simulink library "tqd"  (R2021b)
settings: Solver=VariableStepAuto  StartTime=0.0  StopTime=10.0  RelTol=1e-3
undefined symbols (not defined in the file or in its folder): ATQD_AccelLimitInRange_X_rpm, ATQD_AccelLimitInRange_Y_Nm, ATQD_AccelLimitOvrKi_X_Nm, ATQD_AccelLimitOvrKp_X_Nm, ATQD_BOSMapD_X_rpm, ATQD_BOSMapD_Y_pct, ATQD_BOSMapR_X_rpm, ATQD_BOSMapR_Y_pct, ATQD_HVBCurrSmooth_X_A, ATQD_LHMTqMapDLC_X_rpm, ATQD_LHMTqMapDLC_Y_pct, ATQD_LHMTqMapRLC_X_rpm, ATQD_LHMTqMapRLC_Y_pct, ATQD_NormalMapDLC_X_rpm, ATQD_NormalMapDLC_Y_pct, ATQD_NormalTqDecSR_X_rpm, ATQD_NormalTqDecSR_Y_Nm, ATQD_NormalTqIncSR_X_rpm, ATQD_NormalTqIncSR_Y_Nm, ATQD_OPDMapRLC_X_rpm, ATQD_OPDMapRLC_Y_pct, ATQD_RollRegTorReq_X_rpm, ATQD_RollRegTorReq_Y_enum, ATQD_VehSpdLimitInRange_X_rpm, ATQD_VehSpdLimitInRange_Y_Nm, ATQD_VehSpdLimitOvrKi_X_Nm, ATQD_VehSpdLimitOvrKp_X_Nm, EIGHT_INT, ENUM_BRAKEPEDAL_PRESSED, ENUM_BRAKEPEDAL_RELEASED, ENUM_COMBOKEY_DOWN, ENUM_COMBOKEY_M1, ENUM_COMBOKEY_M2, ENUM_COMBOKEY_NONE, ENUM_COMBOKEY_RKNEE, ENUM_COMBOKEY_STOPLV, ENUM_COMBOKEY_UP, ENUM_CP2VKNEEREQ_REQUEST, ENUM_CP2VNLVREQ_LEVEL1, ENUM_CP2VNLVREQ_LEVEL2, ENUM_CP2VNLVREQ_LOWER, ENUM_CP2VNLVREQ_STOPLV, ENUM_CP2VNLVREQ_UPPER, ENUM_CREEPIND_DISABLE, ENUM_CREEPIND_READY, ENUM_CREEPIND_RUNNING, ENUM_CREEPIND_WARNING, ENUM_DRIVELINERELEASE_RELEASE, ENUM_EBSTORQUERWQ_LIMIT, ENUM_EBSTORQUERWQ_TORQUE, ENUM_ECPVCUDRM_CONFORT, ENUM_ECPVCUDRM_ECO, ENUM_ECPVCUDRM_NORMAL, ENUM_ECPVCUDRM_NOTAVAILABLE, ENUM_EMTqModeDrvBrk_Accel, ENUM_EMTqModeDrvBrk_Brake, ENUM_EMTqModeDrvBrk_Coast, ENUM_ETC2ACTDRIVEDIR_BACKWARD, ENUM_ETC2ACTDRIVEDIR_FORWARD, ENUM_ETC2ACTDRIVEDIR_STILL ... (+341)
libraries: simulink x109, hcu_lib x67
(part 13 of 13)

== stateflow chart tqd/TQD/OutpConvert/Buzzer Request/Combo Key Flasher/Chart ==
  state init
    en:
    time_cnt = ZERO_INT;
    ON_flg = TRUE;
    OFF_flg = FALSE;
    out = FALSE;
    CycleCnt_cnt = FALSE;
  state OFF
    en:
    out = FALSE;
    time_cnt = ZERO_INT;
    OFF -> (junction 38) [order 1]
    (junction 38) -> OFF : {time_cnt = time_cnt + ZERO_INT;}
  state ON
    en:
    out = TRUE;
    time_cnt = ZERO_INT;
    du:
    time_cnt = time_cnt + ONE_INT;
  state WAIT
    en:
    out = FALSE;
    time_cnt = ZERO_INT;
    du:
    time_cnt = time_cnt + ONE_INT;
  (default) -> init
  init -> (junction 57)
  (junction 57) -> ON : [ON_flg && VSCP_FlasherEn_flg]
  OFF -> (junction 46) [order 2] : [time_cnt > OFF_cnt]
  (junction 46) -> (junction 47) : {time_cnt = ZERO_INT;
      |  ON_flg = TRUE;
      |  OFF_flg = FALSE;
      |  CycleCnt_cnt = CycleCnt_cnt +ONE_INT;}
  (junction 47) -> ON : [ON_flg]
  ON -> (junction 44) : [time_cnt > ON_cnt]
  (junction 44) -> (junction 42) : {time_cnt = ZERO_INT;
      |  ON_flg = FALSE;
      |  OFF_flg = TRUE;}
  (junction 42) -> OFF : [OFF_flg]
  OFF -> (junction 66) [order 1] : [time_cnt > OFF_cnt && CycleCnt_cnt >= Cycle_cnt]
  (junction 66) -> WAIT : {time_cnt = ZERO_INT;}
  (junction 62) -> ON : {time_cnt = ZERO_INT;
      |  ON_flg = TRUE;
      |  OFF_flg = FALSE;
      |  CycleCnt_cnt = ZERO_INT;}
  WAIT -> (junction 62) : [time_cnt >= WAIT_cnt && VSCP_FlasherEn_flg]
  data: ON_cnt input; OFF_cnt input; WAIT_cnt input; Cycle_cnt input; out output boolean; time_cnt local uint8; OFF_flg local boolean; ON_flg local boolean; CycleCnt_cnt local uint8; VSCP_FlasherEn_flg input; FALSE parameter; TRUE parameter; ONE_INT parameter; ZERO_INT parameter

== stateflow chart tqd/TQD/OutpConvert/Buzzer Request/Parking Protect Flasher/Chart ==
  state init
    en:
    time_cnt = ZERO_INT;
    ON_flg = TRUE;
    OFF_flg = FALSE;
    out = FALSE;
    CycleCnt_cnt = FALSE;
  state OFF
    en:
    out = FALSE;
    time_cnt = ZERO_INT;
    OFF -> (junction 38) [order 1]
    (junction 38) -> OFF : {time_cnt = time_cnt + ZERO_INT;}
  state ON
    en:
    out = TRUE;
    time_cnt = ZERO_INT;
    du:
    time_cnt = time_cnt + ONE_INT;
  state WAIT
    en:
    out = FALSE;
    time_cnt = ZERO_INT;
    du:
    time_cnt = time_cnt + ONE_INT;
  (default) -> init
  init -> (junction 57)
  (junction 57) -> ON : [ON_flg && VSCP_FlasherEn_flg]
  OFF -> (junction 46) [order 2] : [time_cnt > OFF_cnt]
  (junction 46) -> (junction 47) : {time_cnt = ZERO_INT;
      |  ON_flg = TRUE;
      |  OFF_flg = FALSE;
      |  CycleCnt_cnt = CycleCnt_cnt +ONE_INT;}
  (junction 47) -> ON : [ON_flg]
  ON -> (junction 44) : [time_cnt > ON_cnt]
  (junction 44) -> (junction 42) : {time_cnt = ZERO_INT;
      |  ON_flg = FALSE;
      |  OFF_flg = TRUE;}
  (junction 42) -> OFF : [OFF_flg]
  OFF -> (junction 66) [order 1] : [time_cnt > OFF_cnt && CycleCnt_cnt >= Cycle_cnt]
  (junction 66) -> WAIT : {time_cnt = ZERO_INT;}
  (junction 62) -> ON : {time_cnt = ZERO_INT;
      |  ON_flg = TRUE;
      |  OFF_flg = FALSE;
      |  CycleCnt_cnt = ZERO_INT;}
  WAIT -> (junction 62) : [time_cnt >= WAIT_cnt && VSCP_FlasherEn_flg]
  data: ON_cnt input; OFF_cnt input; WAIT_cnt input; Cycle_cnt input; out output boolean; time_cnt local uint8; OFF_flg local boolean; ON_flg local boolean; CycleCnt_cnt local uint8; VSCP_FlasherEn_flg input; FALSE parameter; TRUE parameter; ONE_INT parameter; ZERO_INT parameter

== stateflow chart tqd/TQD/OutpConvert/Buzzer Request/Power Up Fail Flasher/Chart ==
  state init
    en:
    time_cnt = ZERO_INT;
    ON_flg = TRUE;
    OFF_flg = FALSE;
    out = FALSE;
    CycleCnt_cnt = FALSE;
  state OFF
    en:
    out = FALSE;
    time_cnt = ZERO_INT;
    OFF -> (junction 38) [order 1]
    (junction 38) -> OFF : {time_cnt = time_cnt + ZERO_INT;}
  state ON
    en:
    out = TRUE;
    time_cnt = ZERO_INT;
    du:
    time_cnt = time_cnt + ONE_INT;
  state WAIT
    en:
    out = FALSE;
    time_cnt = ZERO_INT;
    du:
    time_cnt = time_cnt + ONE_INT;
  (default) -> init
  init -> (junction 57)
  (junction 57) -> ON : [ON_flg && VSCP_FlasherEn_flg]
  OFF -> (junction 46) [order 2] : [time_cnt > OFF_cnt]
  (junction 46) -> (junction 47) : {time_cnt = ZERO_INT;
      |  ON_flg = TRUE;
      |  OFF_flg = FALSE;
      |  CycleCnt_cnt = CycleCnt_cnt +ONE_INT;}
  (junction 47) -> ON : [ON_flg]
  ON -> (junction 44) : [time_cnt > ON_cnt]
  (junction 44) -> (junction 42) : {time_cnt = ZERO_INT;
      |  ON_flg = FALSE;
      |  OFF_flg = TRUE;}
  (junction 42) -> OFF : [OFF_flg]
  OFF -> (junction 66) [order 1] : [time_cnt > OFF_cnt && CycleCnt_cnt >= Cycle_cnt]
  (junction 66) -> WAIT : {time_cnt = ZERO_INT;}
  (junction 62) -> ON : {time_cnt = ZERO_INT;
      |  ON_flg = TRUE;
      |  OFF_flg = FALSE;
      |  CycleCnt_cnt = ZERO_INT;}
  WAIT -> (junction 62) : [time_cnt >= WAIT_cnt && VSCP_FlasherEn_flg]
  data: ON_cnt input; OFF_cnt input; WAIT_cnt input; Cycle_cnt input; out output boolean; time_cnt local uint8; OFF_flg local boolean; ON_flg local boolean; CycleCnt_cnt local uint8; VSCP_FlasherEn_flg input; FALSE parameter; TRUE parameter; ONE_INT parameter; ZERO_INT parameter

== stateflow chart tqd/TQD/OutpConvert/Buzzer Request/Power Up Finished Flasher/Chart ==
  state init
    en:
    time_cnt = ZERO_INT;
    ON_flg = TRUE;
    OFF_flg = FALSE;
    out = FALSE;
    CycleCnt_cnt = FALSE;
  state OFF
    en:
    out = FALSE;
    time_cnt = ZERO_INT;
    OFF -> (junction 38) [order 1]
    (junction 38) -> OFF : {time_cnt = time_cnt + ZERO_INT;}
  state ON
    en:
    out = TRUE;
    time_cnt = ZERO_INT;
    du:
    time_cnt = time_cnt + ONE_INT;
  state WAIT
    en:
    out = FALSE;
    time_cnt = ZERO_INT;
    du:
    time_cnt = time_cnt + ONE_INT;
  (default) -> init
  init -> (junction 57)
  (junction 57) -> ON : [ON_flg && VSCP_FlasherEn_flg]
  OFF -> (junction 46) [order 2] : [time_cnt > OFF_cnt]
  (junction 46) -> (junction 47) : {time_cnt = ZERO_INT;
      |  ON_flg = TRUE;
      |  OFF_flg = FALSE;
      |  CycleCnt_cnt = CycleCnt_cnt +ONE_INT;}
  (junction 47) -> ON : [ON_flg]
  ON -> (junction 44) : [time_cnt > ON_cnt]
  (junction 44) -> (junction 42) : {time_cnt = ZERO_INT;
      |  ON_flg = FALSE;
      |  OFF_flg = TRUE;}
  (junction 42) -> OFF : [OFF_flg]
  OFF -> (junction 66) [order 1] : [time_cnt > OFF_cnt && CycleCnt_cnt >= Cycle_cnt]
  (junction 66) -> WAIT : {time_cnt = ZERO_INT;}
  (junction 62) -> ON : {time_cnt = ZERO_INT;
      |  ON_flg = TRUE;
      |  OFF_flg = FALSE;
      |  CycleCnt_cnt = ZERO_INT;}
  WAIT -> (junction 62) : [time_cnt >= WAIT_cnt && VSCP_FlasherEn_flg]
  data: ON_cnt input; OFF_cnt input; WAIT_cnt input; Cycle_cnt input; out output boolean; time_cnt local uint8; OFF_flg local boolean; ON_flg local boolean; CycleCnt_cnt local uint8; VSCP_FlasherEn_flg input; FALSE parameter; TRUE parameter; ONE_INT parameter; ZERO_INT parameter

== stateflow chart tqd/TQD/OutpConvert/Buzzer Request/Power Up Start Flasher/Chart ==
  state init
    en:
    time_cnt = ZERO_INT;
    ON_flg = TRUE;
    OFF_flg = FALSE;
    out = FALSE;
    CycleCnt_cnt = FALSE;
  state OFF
    en:
    out = FALSE;
    time_cnt = ZERO_INT;
    OFF -> (junction 38) [order 1]
    (junction 38) -> OFF : {time_cnt = time_cnt + ZERO_INT;}
  state ON
    en:
    out = TRUE;
    time_cnt = ZERO_INT;
    du:
    time_cnt = time_cnt + ONE_INT;
  state WAIT
    en:
    out = FALSE;
    time_cnt = ZERO_INT;
    du:
    time_cnt = time_cnt + ONE_INT;
  (default) -> init
  init -> (junction 57)
  (junction 57) -> ON : [ON_flg && VSCP_FlasherEn_flg]
  OFF -> (junction 46) [order 2] : [time_cnt > OFF_cnt]
  (junction 46) -> (junction 47) : {time_cnt = ZERO_INT;
      |  ON_flg = TRUE;
      |  OFF_flg = FALSE;
      |  CycleCnt_cnt = CycleCnt_cnt +ONE_INT;}
  (junction 47) -> ON : [ON_flg]
  ON -> (junction 44) : [time_cnt > ON_cnt]
  (junction 44) -> (junction 42) : {time_cnt = ZERO_INT;
      |  ON_flg = FALSE;
      |  OFF_flg = TRUE;}
  (junction 42) -> OFF : [OFF_flg]
  OFF -> (junction 66) [order 1] : [time_cnt > OFF_cnt && CycleCnt_cnt >= Cycle_cnt]
  (junction 66) -> WAIT : {time_cnt = ZERO_INT;}
  (junction 62) -> ON : {time_cnt = ZERO_INT;
      |  ON_flg = TRUE;
      |  OFF_flg = FALSE;
      |  CycleCnt_cnt = ZERO_INT;}
  WAIT -> (junction 62) : [time_cnt >= WAIT_cnt && VSCP_FlasherEn_flg]
  data: ON_cnt input; OFF_cnt input; WAIT_cnt input; Cycle_cnt input; out output boolean; time_cnt local uint8; OFF_flg local boolean; ON_flg local boolean; CycleCnt_cnt local uint8; VSCP_FlasherEn_flg input; FALSE parameter; TRUE parameter; ONE_INT parameter; ZERO_INT parameter

== stateflow chart tqd/TQD/Input_Convert/Function/TUpA/TUpAStatus ==
  state Disable
    en:
    VTQD_TUpAIND_enum = ENUM_TUPAIND_DISABLE;
    VTQD_VCUEBSHHSw_enum = ENUM_VCUEBSHHSW_OFF;
    VTQD_VCUEBSRd4BR_enum = ENUM_VCUEBSRD4BR_NOTREADY;
    VTQD_TUpADisableCreep_flg = FALSE;
    VTQD_TUpAReadyReset_flg = FALSE;
  state Ready
    en:
    VTQD_TUpAIND_enum = ENUM_TUPAIND_READY;
  state EnableCheck
    en:
    VTQD_VCUEBSHHSw_enum = ENUM_VCUEBSHHSW_ON;
    VTQD_TUpADisableCreep_flg = TRUE;
    VTQD_HHActive_flg = FALSE;
    VTQD_HHActiveTimeout_flg = FALSE;
    VTQD_TUpAReadyReset_flg = TRUE;
    (default) -> (junction 8) : {
        | VTQD_HHActiveTime_s = ZERO_FLOAT;
        | }
    EnableCheck -> (junction 8) [order 1]
    (junction 8) -> (junction 10) [order 1] : [VINP_HillHolderMode_enum == ENUM_HHMODE_ACTIVE]
    (junction 8) -> (junction 14) [order 2] : {
        | VTQD_HHActiveTime_s += task_time_s;
        | }
    (junction 10) -> (junction 12) : {
        | VTQD_HHActive_flg = TRUE;
        |  }
    (junction 14) -> (junction 107) [order 1] : [VTQD_HHActiveTime_s > KTQD_TUpAHHFbkTO_s]
    (junction 14) -> (junction 111) [order 2]
    (junction 107) -> (junction 109) : {
        | VTQD_HHActiveTimeout_flg = TRUE;
        | }
    (junction 109) -> (junction 111)
    (junction 12) -> (junction 109)
  state Warning
    en:
    VTQD_TUpAIND_enum = ENUM_TUPAIND_WARNING;
  state RUN
    en:
    VTQD_TUpAIND_enum = ENUM_TUPAIND_RUNNING;
    VTQD_HHDeactiveWarn_flg = FALSE;
    (default) -> (junction 115)
    RUN -> (junction 115) [order 1]
    (junction 115) -> (junction 117) [order 1] : [VINP_HillHolderMode_enum ~= ENUM_HHMODE_ACTIVE]
    (junction 115) -> (junction 121) [order 2]
    (junction 117) -> (junction 119) : {
        | VTQD_HHDeactiveWarn_flg = TRUE;
        | }
    (junction 119) -> (junction 121)
  state DisableCheck
    en:
    VTQD_VCUEBSHHSw_enum = ENUM_VCUEBSHHSW_OFF;
    VTQD_VCUEBSRd4BR_enum = ENUM_VCUEBSRD4BR_READY;
    VTQD_HHDeactive_flg = FALSE;
    (default) -> (junction 38) : {
        | VTQD_HHDisableTime_s = ZERO_FLOAT;
        | }
    DisableCheck -> (junction 38) [order 1]
    (junction 38) -> (junction 44) [order 1] : [VINP_HillHolderMode_enum == ENUM_HHMODE_INACTIVE]
    (junction 38) -> (junction 42) [order 2] : {
        | VTQD_HHDisableTime_s += task_time_s;
        | }
    (junction 44) -> (junction 40) : {
        | VTQD_HHDeactive_flg = TRUE;
        |  }
    (junction 40) -> (junction 42)
  state SignalReset
    en:
    VTQD_VCUEBSHHSw_enum = ENUM_VCUEBSHHSW_OFF;
    VTQD_VCUEBSRd4BR_enum = ENUM_VCUEBSRD4BR_NOTREADY;
    VTQD_TUpADisableCreep_flg = FALSE;
    VTQD_Warn2Disable_flg = FALSE;
    (default) -> (junction 163) : {
        | VTQD_TUpAWarnTime = ZERO_FLOAT;
        | }
    SignalReset -> (junction 163) [order 1]
    (junction 163) -> (junction 164) [order 1] : [VTQD_TUpAIND_enum == ENUM_TUPAIND_WARNING]
    (junction 164) -> (junction 165) : {
        | VTQD_TUpAWarnTime += task_time_s;
        | }
    (junction 163) -> (junction 167) [order 2]
    (junction 165) -> (junction 166) : [VTQD_TUpAWarnTime > KTQD_TUpAWarnLatchTime_s]
    (junction 166) -> (junction 171) : {
        | VTQD_Warn2Disable_flg = TRUE;
        | }
    (junction 167) -> (junction 168) [order 1] : [VTQD_TUpAIND_enum == ENUM_TUPAIND_RUNNING]
    (junction 167) -> (junction 169) [order 2]
    (junction 168) -> (junction 170) : {
        | VTQD_Warn2Disable_flg = TRUE;
        | }
    (junction 170) -> (junction 169)
    (junction 171) -> (junction 170)
  (default) -> Disable
  (junction 63) -> Disable
  Disable -> (junction 187) [order 2] : [VDMM_DTCPBWireFailure_flg]
  (junction 61) -> (junction 63)
  (junction 187) -> Warning
  Ready -> Disable [order 2] : [!VTQD_TUpAReady_flg]
  Disable -> Ready [order 1] : [VTQD_TUpAReady_flg]
  Ready -> EnableCheck [order 1] : [VTQD_TUpAEnableReq_flg]
  EnableCheck -> Warning [order 2] : [VTQD_HHActiveTimeout_flg]
  EnableCheck -> RUN [order 1] : [VTQD_HHActive_flg]
  Warning -> (junction 184) [order 3]
  (junction 33) -> Warning
  Warning -> (junction 68) [order 1]
  Warning -> (junction 104) [order 2]
  (junction 184) -> RUN : [VINP_HillHolderMode_enum == ENUM_HHMODE_ACTIVE]
  RUN -> (junction 33) [order 1] : [VTQD_HHDeactiveWarn_flg]
  RUN -> DisableCheck [order 2] : [VTQD_TUpADisableReq_flg]
  DisableCheck -> SignalReset [order 1] : [VTQD_HHDeactive_flg || VTQD_HHDisableTime_s > KTQD_TUpAHHFbkTO_s]
  (junction 68) -> SignalReset : [VTQD_HHDeactiveWarn_flg &&...
      | VINP_ASRHillHolderSw_enum == ENUM_HHSW_INACTIVE]
  SignalReset -> (junction 61) [order 1] : [(VINP_EBSBrakeSw_enum == ENUM_BRAKEPEDAL_PRESSED ||...
      | VINP_ParkBreakSW_flg ||...
      | VTQD_CreepIND_enum == ENUM_CREEPIND_RUNNING ||...
      | VDHP_AccelPedalDepressed_flg) && VTQD_Warn2Disable_flg]
  (junction 104) -> SignalReset : [VTQD_HHActiveTimeout_flg]
  data: KTQD_TUpAWarnLatchTime_s input; KTQD_TUpAHHFbkTO_s input; VINP_EBSBrakeSw_enum input; VINP_HillHolderMode_enum input; VINP_ParkBreakSW_flg input; VTQD_CreepIND_enum input; VTQD_TUpADisableReq_flg input; VTQD_TUpAEnableReq_flg input; VTQD_TUpAReady_flg input; task_time_s input; VTQD_TUpADisableCreep_flg output boolean; VTQD_TUpAIND_enum output uint8; VTQD_VCUEBSHHSw_enum output uint8; VTQD_VCUEBSRd4BR_enum output uint8; VTQD_HHActiveTime_s local single; VTQD_HHActive_flg local boolean; VTQD_HHDeactive_flg local boolean; VTQD_HHDisableTime_s local single; ENUM_BRAKEPEDAL_PRESSED parameter; ENUM_CREEPIND_RUNNING parameter; ENUM_HHMODE_ACTIVE parameter; ENUM_HHMODE_INACTIVE parameter; ENUM_TUPAIND_DISABLE parameter; ENUM_TUPAIND_READY parameter; ENUM_TUPAIND_RUNNING parameter; ENUM_TUPAIND_WARNING parameter; ENUM_VCUEBSHHSW_OFF parameter; ENUM_VCUEBSRD4BR_NOTREADY parameter; FALSE parameter; TRUE parameter; ENUM_VCUEBSHHSW_ON parameter; ENUM_VCUEBSRD4BR_READY parameter; VINP_ASRHillHolderSw_enum input; VTQD_HHActiveTimeout_flg local boolean; VTQD_HHDeactiveWarn_flg local boolean; ENUM_HHSW_INACTIVE parameter; VDHP_AccelPedalDepressed_flg input; VTQD_TUpAWarnTime local single; VTQD_Warn2Disable_flg local boolean; VTQD_TUpAReadyReset_flg output boolean; VDMM_DTCPBWireFailure_flg input; ZERO_FLOAT parameter

== stateflow chart tqd/TQD/Input_Convert/Function/Ramp Parameter/Ramp Parameter Determination ==
  (default) -> (junction 3)
  (junction 3) -> (junction 30) [order 1] : [VTQD_TqSource_enum == ENUM_TQSOURCE_ESC]
  (junction 3) -> (junction 34) [order 2]
  (junction 30) -> (junction 32) : {
      | VTQD_RampTs_c = KTQD_ESCEnableTs_c;
      | VTQD_RampTqIncSR_Nm = KTQD_ESCEnableIncSR_c;
      | VTQD_RampTqDecSR_Nm = KTQD_ESCEnableDecSR_c;
      | }
  (junction 34) -> (junction 36) [order 1] : [VTQD_POSNEGCONVSM_flg]
  (junction 36) -> (junction 43) [order 1] : [VTQD_ActDriveMode_enum == ENUM_ECPVCUDRM_NORMAL]
  (junction 34) -> (junction 73) [order 2]
  (junction 36) -> (junction 41) [order 2]
  (junction 43) -> (junction 45) : {
      | VTQD_RampTs_c = KTQD_POSNEGSWTs_c;
      | VTQD_RampTqIncSR_Nm = VTQD_NormalTqIncSR_Nm;
      | VTQD_RampTqDecSR_Nm = VTQD_NormalTqDecSR_Nm;
      | }
  (junction 41) -> (junction 49) [order 1] : [VTQD_ActDriveMode_enum == ENUM_ECPVCUDRM_ECO]
  (junction 41) -> (junction 47) [order 2]
  (junction 49) -> (junction 51) : {
      | VTQD_RampTs_c = KTQD_POSNEGSWTs_c;
      | VTQD_RampTqIncSR_Nm = VTQD_ECOTqIncSR_Nm;
      | VTQD_RampTqDecSR_Nm = VTQD_ECOTqDecSR_Nm;
      | }
  (junction 47) -> (junction 53) [order 1] : [VTQD_ActDriveMode_enum == ENUM_ECPVCUDRM_CONFORT]
  (junction 47) -> (junction 58) [order 2] : {
      | VTQD_RampTs_c = KTQD_POSNEGSWTs_c;
      | VTQD_RampTqIncSR_Nm = VTQD_NormalTqIncSR_Nm;
      | VTQD_RampTqDecSR_Nm = VTQD_NormalTqDecSR_Nm;
      | }
  (junction 53) -> (junction 56) : {
      | VTQD_RampTs_c = KTQD_POSNEGSWTs_c;
      | VTQD_RampTqIncSR_Nm = VTQD_ConfortTqIncSR_Nm;
      | VTQD_RampTqDecSR_Nm = VTQD_ConfortTqDecSR_Nm;
      | }
  (junction 73) -> (junction 68) [order 1] : [VTQD_ActDriveMode_enum == ENUM_ECPVCUDRM_NORMAL]
  (junction 73) -> (junction 69) [order 2]
  (junction 68) -> (junction 77) : {
      | VTQD_RampTs_c = KTQD_NormalTs_c;
      | VTQD_RampTqIncSR_Nm = VTQD_NormalTqIncSR_Nm;
      | VTQD_RampTqDecSR_Nm = VTQD_NormalTqDecSR_Nm;
      | }
  (junction 69) -> (junction 66) [order 1] : [VTQD_ActDriveMode_enum == ENUM_ECPVCUDRM_ECO]
  (junction 69) -> (junction 78) [order 2]
  (junction 66) -> (junction 67) : {
      | VTQD_RampTs_c = KTQD_ECOTs_c;
      | VTQD_RampTqIncSR_Nm = VTQD_ECOTqIncSR_Nm;
      | VTQD_RampTqDecSR_Nm = VTQD_ECOTqDecSR_Nm;
      | }
  (junction 78) -> (junction 71) [order 1] : [VTQD_ActDriveMode_enum == ENUM_ECPVCUDRM_CONFORT]
  (junction 78) -> (junction 62) [order 2] : {
      | VTQD_RampTs_c = KTQD_NormalTs_c;
      | VTQD_RampTqIncSR_Nm = VTQD_NormalTqIncSR_Nm;
      | VTQD_RampTqDecSR_Nm = VTQD_NormalTqDecSR_Nm;
      | }
  (junction 71) -> (junction 65) : {
      | VTQD_RampTs_c = KTQD_ConfortTs_c;
      | VTQD_RampTqIncSR_Nm = VTQD_ConfortTqIncSR_Nm;
      | VTQD_RampTqDecSR_Nm = VTQD_ConfortTqDecSR_Nm;
      | }
  data: VTQD_RampTs_c output; VTQD_RampTqIncSR_Nm output; VTQD_TqSource_enum input; ENUM_TQSOURCE_ESC parameter; KTQD_ESCEnableTs_c parameter; KTQD_ESCEnableIncSR_c parameter; KTQD_ESCEnableDecSR_c parameter; VTQD_RampTqDecSR_Nm output; VTQD_POSNEGCONVSM_flg input; KTQD_POSNEGSWTs_c parameter; VTQD_ActDriveMode_enum input; ENUM_ECPVCUDRM_NORMAL parameter; ENUM_ECPVCUDRM_ECO parameter; ENUM_ECPVCUDRM_CONFORT parameter; VTQD_NormalTqIncSR_Nm input; VTQD_NormalTqDecSR_Nm input; VTQD_ECOTqIncSR_Nm input; VTQD_ECOTqDecSR_Nm input; VTQD_ConfortTqIncSR_Nm input; VTQD_ConfortTqDecSR_Nm input; KTQD_NormalTs_c parameter; KTQD_ECOTs_c parameter; KTQD_ConfortTs_c parameter

== stateflow chart tqd/TQD/Input_Convert/Function/Pedal Torque/Torque Command Determination ==
  state Standby
    du:
    VTQD_PedalMapTq_Nm = ZERO_FLOAT;
  state Ready
    (default) -> (junction 30)
    Ready -> (junction 30) [order 1]
    (junction 30) -> (junction 32) [order 1] : [VDHP_LHMRestrictDrivePwr_flg]
    (junction 32) -> (junction 34) [order 1] : [VTQD_GearActualPosn_enum == ENUM_GEARACTUALPOSN_R]
    (junction 30) -> (junction 41) [order 2]
    (junction 32) -> (junction 36) [order 2] : {VTQD_PedalMapTq_Nm = VTQD_LHMTqMapD_Nm;}
    (junction 34) -> (junction 39) : {VTQD_PedalMapTq_Nm = VTQD_LHMTqMapRLC_Nm;}
    (junction 41) -> (junction 43) [order 1] : [VTQD_GearActualPosn_enum == ENUM_GEARACTUALPOSN_R]
    (junction 41) -> (junction 47) [order 2]
    (junction 43) -> (junction 45) : {VTQD_PedalMapTq_Nm = VTQD_OPDMapRLC_Nm;}
    (junction 47) -> (junction 49) [order 1] : [VTQD_ActDriveMode_enum == ENUM_ECPVCUDRM_NORMAL]
    (junction 47) -> (junction 57) [order 2]
    (junction 49) -> (junction 50) : {VTQD_PedalMapTq_Nm = VTQD_NormalTqMapD_Nm;}
    (junction 57) -> (junction 59) [order 1] : [VTQD_ActDriveMode_enum == ENUM_ECPVCUDRM_ECO]
    (junction 57) -> (junction 64) [order 2]
    (junction 59) -> (junction 61) : {VTQD_PedalMapTq_Nm = VTQD_ECOTqMapD_Nm;}
    (junction 64) -> (junction 66) [order 1] : [VTQD_ActDriveMode_enum == ENUM_ECPVCUDRM_CONFORT]
    (junction 64) -> (junction 70) [order 2] : {VTQD_PedalMapTq_Nm = VTQD_NormalTqMapD_Nm;}
    (junction 66) -> (junction 68) : {VTQD_PedalMapTq_Nm = VTQD_ConfortTqMapD_Nm;}
  (default) -> Standby
  Standby -> Ready : [VTQD_GearActualPosn_enum == ENUM_GEARACTUALPOSN_D || ...
      |  VTQD_GearActualPosn_enum == ENUM_GEARACTUALPOSN_R]
  Ready -> Standby [order 1] : [VTQD_GearActualPosn_enum ~= ENUM_GEARACTUALPOSN_D && ...
      |  VTQD_GearActualPosn_enum ~= ENUM_GEARACTUALPOSN_R]
  data: VTQD_GearActualPosn_enum input; VTQD_ActDriveMode_enum input; VDHP_LHMRestrictDrivePwr_flg input; VTQD_NormalTqMapD_Nm input; VTQD_ECOTqMapD_Nm input; VTQD_ConfortTqMapD_Nm input; VTQD_OPDMapRLC_Nm input; VTQD_LHMTqMapRLC_Nm input; VTQD_LHMTqMapD_Nm input; VTQD_PedalMapTq_Nm output single; ZERO_FLOAT parameter; ENUM_GEARACTUALPOSN_D parameter; ENUM_GEARACTUALPOSN_R parameter; ENUM_ECPVCUDRM_NORMAL parameter; ENUM_ECPVCUDRM_ECO parameter; ENUM_ECPVCUDRM_CONFORT parameter

== stateflow chart tqd/TQD/Input_Convert/Function/Shift Modul/Determine_Actual_Gear_Position ==
  state ADASMode
    state Initialize
      (default) -> (junction 387) : {
          | VTQD_InitializeTime_s = 0;
          | VTQD_ParkingPawlPwrOn_flg = FALSE;
          | }
      ADASMode.Initialize -> (junction 387) [order 1]
      (junction 387) -> (junction 385) : {VTQD_InitializeTime_s = VTQD_InitializeTime_s + task_time_s;}
    state ParkingPawlOperate
      (default) -> (junction 163) : {
          | VTQD_ParkingPawlLockTime_s=0;
          | VTQD_ParkingPawlUnlockTime_s=0;
          | VTQD_ParkingPawlLockTimeOut_flg = FALSE;
          | VTQD_ParkingPawlUnlockTimeOut_flg = FALSE;
          | VTQD_ParkingPawlPwrOn_flg = TRUE;
          | VTQD_PTLock_flg = FALSE;
          | VTQD_PTUnlock_flg = FALSE;
          | }
      ADASMode.ParkingPawlOperate -> (junction 163) [order 1]
      (junction 163) -> (junction 164) [order 1] : [(VTQD_GearShiftPosn_enum == ENUM_GEARSHIFTPOSN_P)]
      (junction 163) -> (junction 263) [order 2]
      (junction 164) -> (junction 167) : {
          | VTQD_ParkingPawlEnable_flg = TRUE;
          | }
      (junction 263) -> (junction 166) [order 1] : [(VTQD_GearShiftPosn_enum ~= ENUM_GEARSHIFTPOSN_P)]
      (junction 263) -> (junction 173) [order 2]
      (junction 166) -> (junction 169) : {
          | VTQD_ParkingPawlEnable_flg = FALSE;
          | }
      (junction 169) -> (junction 170) [order 1] : [!VINP_ParkingPawlLock_flg]
      (junction 169) -> (junction 255) [order 2] : {
          | VTQD_ParkingPawlUnlockTime_s += task_time_s;
          | }
      (junction 170) -> (junction 176) : {
          | VTQD_PTUnlock_flg = TRUE;
          | }
      (junction 167) -> (junction 168) [order 1] : [VINP_ParkingPawlLock_flg]
      (junction 167) -> (junction 248) [order 2] : {
          | VTQD_ParkingPawlLockTime_s += task_time_s;
          | }
      (junction 168) -> (junction 178) : {
          | VTQD_PTLock_flg = TRUE;
          | }
      (junction 255) -> (junction 257) [order 1] : [VTQD_ParkingPawUnlockTime_s >= KTQD_RotateShiftMaxTime_s]
      (junction 255) -> (junction 175) [order 2]
      (junction 257) -> (junction 260) : {
          | VTQD_ParkingPawlUnlockTimeOut_flg = TRUE;
          | }
      (junction 248) -> (junction 250) [order 1] : [VTQD_ParkingPawLockTime_s >= KTQD_RotateShiftMaxTime_s]
      (junction 248) -> (junction 177) [order 2]
      (junction 250) -> (junction 252) : {
          | VTQD_ParkingPawlLockTimeOut_flg = TRUE;
          | }
      (junction 175) -> (junction 173)
      (junction 260) -> (junction 175)
      (junction 177) -> (junction 176)
      (junction 252) -> (junction 177)
      (junction 176) -> (junction 260)
      (junction 178) -> (junction 252)
    state P
      en:
      VTQD_GearActualPosn_enum = ENUM_GEARACTUALPOSN_P;
      %VTQD_TMRotateDirectionReq_enum = ENUM_TMROTATEDIRECTREQ_NONE;
      VTQD_ParkingPawlPwrOn_flg = TRUE;
      VTQD_ParkingPawlEnable_flg = TRUE;
    state N
      en:
      VTQD_GearActualPosn_enum = ENUM_GEARACTUALPOSN_N;
      %VTQD_TMRotateDirectionReq_enum = ENUM_TMROTATEDIRECTREQ_NONE;
      VTQD_ParkingPawlPwrOn_flg = TRUE;
      VTQD_ParkingPawlEnable_flg = FALSE;
    state D
      en:
      VTQD_GearActualPosn_enum = ENUM_GEARACTUALPOSN_D;
      %VTQD_TMRotateDirectionReq_enum = ENUM_TMROTATEDIRECTREQ_FWD;
      VTQD_ParkingPawlPwrOn_flg = TRUE;
      VTQD_ParkingPawlEnable_flg = FALSE;
    state R
      en:
      VTQD_GearActualPosn_enum = ENUM_GEARACTUALPOSN_R;
      %VTQD_TMRotateDirectionReq_enum = ENUM_TMROTATEDIRECTREQ_REV;
      VTQD_ParkingPawlPwrOn_flg = TRUE;
      VTQD_ParkingPawlEnable_flg = FALSE;
    (default) -> ADASMode.Initialize
    ADASMode.Initialize -> (junction 268) [order 1] : [(VTQD_InitializeTime_s > KTQD_InitializeWaitTime4ADAS_s)]
    (junction 268) -> ADASMode.ParkingPawlOperate
    ADASMode.P -> ADASMode.ParkingPawlOperate : [VTQD_RNDTrig_flg]
    ADASMode.ParkingPawlOperate -> ADASMode.P [order 1] : [(VTQD_ParkingPawlUnlockTimeOut_flg || VTQD_PTLock_flg)]
    ADASMode.ParkingPawlOperate -> (junction 245) [order 2]
    (junction 215) -> ADASMode.ParkingPawlOperate
    (junction 213) -> ADASMode.ParkingPawlOperate
    ADASMode.ParkingPawlOperate -> (junction 212) [order 3]
    (junction 216) -> ADASMode.ParkingPawlOperate
    ADASMode.ParkingPawlOperate -> (junction 219) [order 4]
    (junction 245) -> ADASMode.N : [(VTQD_GearShiftPosn_enum == ENUM_GEARSHIFTPOSN_N && VTQD_PTUnlock_flg)||...
        |  (VTQD_ParkingPawlLockTimeOut_flg)]
    (junction 246) -> ADASMode.N
    (junction 218) -> (junction 246)
    ADASMode.N -> (junction 153) [order 3] : [(VTQD_GearShiftPosn_enum == ENUM_GEARSHIFTPOSN_R)]
    ADASMode.N -> (junction 215) [order 1] : [(VTQD_GearShiftPosn_enum == ENUM_GEARSHIFTPOSN_P)]
    (junction 153) -> (junction 214)
    ADASMode.N -> ADASMode.D [order 2] : [(VTQD_GearShiftPosn_enum == ENUM_GEARSHIFTPOSN_D)]
    ADASMode.D -> ADASMode.N [order 2] : [(VTQD_GearShiftPosn_enum == ENUM_GEARSHIFTPOSN_N)]
    ADASMode.D -> (junction 213) [order 3] : [(VTQD_GearShiftPosn_enum == ENUM_GEARSHIFTPOSN_P)]
    (junction 212) -> ADASMode.D : [(VTQD_GearShiftPosn_enum == ENUM_GEARSHIFTPOSN_D && VTQD_PTUnlock_flg)]
    ADASMode.D -> ADASMode.R [order 1] : [(VTQD_GearShiftPosn_enum == ENUM_GEARSHIFTPOSN_R)]
    ADASMode.R -> ADASMode.D [order 1] : [(VTQD_GearShiftPosn_enum == ENUM_GEARSHIFTPOSN_D)]
    (junction 214) -> ADASMode.R
    ADASMode.R -> (junction 216) [order 2] : [(VTQD_GearShiftPosn_enum == ENUM_GEARSHIFTPOSN_P)]
    ADASMode.R -> (junction 218) [order 3] : [(VTQD_GearShiftPosn_enum == ENUM_GEARSHIFTPOSN_N)]
    (junction 219) -> ADASMode.R : [(VTQD_GearShiftPosn_enum == ENUM_GEARSHIFTPOSN_R && VTQD_PTUnlock_flg)]
  state NormalMode
    state ParkingPawlOperate
      (default) -> (junction 285) : {
          | VTQD_ParkingPawlLockTime_s=0;
          | VTQD_ParkingPawlUnlockTime_s=0;
          | VTQD_ParkingPawlLockTimeOut_flg = FALSE;
          | VTQD_ParkingPawlUnlockTimeOut_flg = FALSE;
          | VTQD_ParkingPawlPwrOn_flg = TRUE;
          | VTQD_PTLock_flg = FALSE;
          | VTQD_PTUnlock_flg = FALSE;
          | }
      NormalMode.ParkingPawlOperate -> (junction 285) [order 1]
      (junction 285) -> (junction 286) [order 1] : [VTQD_GearShiftPosn_enum == ENUM_GEARSHIFTPOSN_P]
      (junction 286) -> (junction 291) : {
          | VTQD_ParkingPawlEnable_flg = TRUE;
          | }
      (junction 285) -> (junction 288) [order 2]
      (junction 288) -> (junction 287) [order 1] : [VTQD_GearShiftPosn_enum != ENUM_GEARSHIFTPOSN_P]
      (junction 288) -> (junction 297) [order 2]
      (junction 287) -> (junction 289) : {
          | VTQD_ParkingPawlEnable_flg = FALSE;
          | }
      (junction 289) -> (junction 290) [order 1] : [!VINP_ParkingPawlLock_flg]
      (junction 289) -> (junction 293) [order 2] : {
          | VTQD_ParkingPawlUnlockTime_s += task_time_s;
          | }
      (junction 290) -> (junction 299) : {
          | VTQD_PTUnlock_flg = TRUE;
          | }
      (junction 291) -> (junction 292) [order 1] : [VINP_ParkingPawlLock_flg]
      (junction 291) -> (junction 295) [order 2] : {
          | VTQD_ParkingPawlLockTime_s += task_time_s;
          | }
      (junction 292) -> (junction 301) : {
          | VTQD_PTLock_flg = TRUE;
          | }
      (junction 293) -> (junction 294) [order 1] : [VTQD_ParkingPawUnlockTime_s >= KTQD_RotateShiftMaxTime_s]
      (junction 293) -> (junction 298) [order 2]
      (junction 294) -> (junction 302) : {
          | VTQD_ParkingPawlUnlockTimeOut_flg = TRUE;
          | }
      (junction 295) -> (junction 296) [order 1] : [VTQD_ParkingPawLockTime_s >= KTQD_RotateShiftMaxTime_s]
      (junction 295) -> (junction 300) [order 2]
      (junction 296) -> (junction 303) : {
          | VTQD_ParkingPawlLockTimeOut_flg = TRUE;
          | }
      (junction 302) -> (junction 298)
      (junction 300) -> (junction 299)
      (junction 303) -> (junction 300)
      (junction 298) -> (junction 297)
      (junction 299) -> (junction 302)
      (junction 301) -> (junction 303)
    state Initialize
      (default) -> (junction 66) : {
          | VTQD_InitializeTime_s = 0;
          | VTQD_ParkingPawlPwrOn_flg = FALSE;
          | }
      NormalMode.Initialize -> (junction 66) [order 1]
      (junction 66) -> (junction 73) : {VTQD_InitializeTime_s = VTQD_InitializeTime_s + task_time_s;}
    state P
      en:
      VTQD_GearActualPosn_enum = ENUM_GEARACTUALPOSN_P;
      %VTQD_TMRotateDirectionReq_enum = ENUM_TMROTATEDIRECTREQ_NONE;
      VTQD_ParkingPawlPwrOn_flg = TRUE;
      VTQD_ParkingPawlEnable_flg = TRUE;
    state N
      en:
      VTQD_GearActualPosn_enum = ENUM_GEARACTUALPOSN_N;
      %VTQD_TMRotateDirectionReq_enum = ENUM_TMROTATEDIRECTREQ_NONE;
      VTQD_ParkingPawlPwrOn_flg = TRUE;
      VTQD_ParkingPawlEnable_flg = FALSE;
    state AutoP
      en:
      VTQD_GearActualPosn_enum = ENUM_GEARACTUALPOSN_D;
      %VTQD_TMRotateDirectionReq_enum = ENUM_TMROTATEDIRECTREQ_FWD;
      VTQD_ParkingPawlPwrOn_flg = TRUE;
      VTQD_ParkingPawlEnable_flg = TRUE;
      (default) -> (junction 341) : {
          | VTQD_ParkingPawlLockTime_s=0;
          | VTQD_ParkingPawlUnlockTime_s=0;
          | VTQD_ParkingPawlLockTimeOut_flg = FALSE;
          | VTQD_ParkingPawlUnlockTimeOut_flg = FALSE;
          | VTQD_ParkingPawlPwrOn_flg = TRUE;
          | VTQD_PTLock_flg = FALSE;
          | VTQD_PTUnlock_flg = FALSE;
          | }
      AutoP -> (junction 341) [order 1]
      (junction 341) -> (junction 352)
      (junction 352) -> (junction 333) [order 1] : [(!VTQD_AutoPark_flg)||...
          |  (VTQD_GearShiftPosn_enum == ENUM_GEARSHIFTPOSN_N)||...
          |  (VTQD_GearShiftPosn_enum == ENUM_GEARSHIFTPOSN_R)]
      (junction 352) -> (junction 338) [order 2]
      (junction 333) -> (junction 346) : {
          | VTQD_ParkingPawlEnable_flg = FALSE;
          | }
      (junction 346) -> (junction 334) [order 1] : [!VINP_ParkingPawlLock_flg]
      (junction 346) -> (junction 339) [order 2] : {
          | VTQD_ParkingPawlUnlockTime_s += task_time_s;
          | }
      (junction 334) -> (junction 340) : {
          | VTQD_PTUnlock_flg = TRUE;
          | }
      (junction 339) -> (junction 337) [order 1] : [VTQD_ParkingPawUnlockTime_s >= KTQD_RotateShiftMaxTime_s]
      (junction 339) -> (junction 347) [order 2]
      (junction 337) -> (junction 348) : {
          | VTQD_ParkingPawlUnlockTimeOut_flg = TRUE;
          | }
      (junction 347) -> (junction 338)
      (junction 348) -> (junction 347)
      (junction 340) -> (junction 348)
    state D
      en:
      VTQD_GearActualPosn_enum = ENUM_GEARACTUALPOSN_D;
      %VTQD_TMRotateDirectionReq_enum = ENUM_TMROTATEDIRECTREQ_FWD;
      VTQD_ParkingPawlPwrOn_flg = TRUE;
      VTQD_ParkingPawlEnable_flg = FALSE;
    state R
      en:
      VTQD_GearActualPosn_enum = ENUM_GEARACTUALPOSN_R;
      %VTQD_TMRotateDirectionReq_enum = ENUM_TMROTATEDIRECTREQ_REV;
      VTQD_ParkingPawlPwrOn_flg = TRUE;
      VTQD_ParkingPawlEnable_flg = FALSE;
    (default) -> NormalMode.Initialize
    NormalMode.P -> NormalMode.ParkingPawlOperate : [(VTQD_RNDTrig_flg)&&(VINP_BrkSwOn_flg)&&(VPSA_IGNActive_flg)]
    NormalMode.Initialize -> NormalMode.P [order 1] : [(VPSA_IGNActive_flg)&&(VTQD_InitializeTime_s > KTQD_InitializeWaitTime_s)&&...
        | (VTQD_GearShiftPosn_enum == ENUM_GEARSHIFTPOSN_P)]
    NormalMode.ParkingPawlOperate -> NormalMode.P [order 1] : [(VTQD_PTLock_flg || VTQD_ParkingPawlUnlockTimeOut_flg)]
    NormalMode.Initialize -> (junction 273) [order 2]
    NormalMode.ParkingPawlOperate -> (junction 71) [order 2]
    (junction 81) -> NormalMode.ParkingPawlOperate
    (junction 382) -> NormalMode.ParkingPawlOperate
    (junction 88) -> NormalMode.ParkingPawlOperate
    NormalMode.ParkingPawlOperate -> (junction 93) [order 3]
    (junction 89) -> NormalMode.ParkingPawlOperate
    NormalMode.ParkingPawlOperate -> (junction 94) [order 4]
    (junction 273) -> NormalMode.N : [((VPSA_IGNActive_flg)&&(VTQD_InitializeTime_s > KTQD_InitializeWaitTime_s)) ||...
        |  (VTQD_ADASModeDisact_flg)]
    (junction 71) -> NormalMode.N : [(VTQD_GearShiftPosn_enum == ENUM_GEARSHIFTPOSN_N && VTQD_PTUnlock_flg)||...
        |  (VTQD_ParkingPawlLockTimeOut_flg)]
    (junction 75) -> NormalMode.N
    (junction 78) -> (junction 75)
    NormalMode.N -> (junction 81) [order 1] : [(VTQD_GearShiftPosn_enum == ENUM_GEARSHIFTPOSN_P)&&...
        | (VINP_VehSpd_kph<=KTQD_GearShiftPSpd_kph)&& (VPSA_IGNActive_flg)]
    NormalMode.N -> (junction 91) [order 3] : [(VTQD_GearShiftPosn_enum == ENUM_GEARSHIFTPOSN_R && VFUN_EVDriveReady_flg ...
        |   && !VSCP_GearFlashInd_flg && !VTQD_DMSLossLimitGear_flg && !VDMM_DTCDMSRCIncorrect_flg...
        |   && ((VINP_BrkSwOn_flg && VINP_VehSpd_kph<=KTQD_GearShiftRAllowSpd_kph &&...
        |  abs(VINP_TMSpd_rpm) <= KTQD_GearShiftRAllowTMSpd_rpm)||...
        |    (VINP_VehSpd_kph > KTQD_GearShiftRAllowSpd_kph && ...
        |     VSCP_EVCU1VehActDrvDir_enum ~= ENUM_VEHACTDRVDIR_FORWARD)))]
    (junction 91) -> (junction 90)
    NormalMode.D -> NormalMode.N [order 2] : [ VTQD_GearShiftPosn_enum == ENUM_GEARSHIFTPOSN_N || ...
        |   (!VFUN_EVDriveReady_flg) || (VTQD_GearShiftPosn_enum == ENUM_GEARSHIFTPOSN_INVALID) || ...
        |    VSCP_GearFlashInd_flg || ...
        |   (VTQD_DMSLossLimitGear_flg && VINP_VehSpd_kph<=KTQD_DMSLostTorqLimit_kph) || ...
        | (VDMM_DTCDMSRCIncorrect_flg && VINP_ParkBrakeSW_flg)]
    NormalMode.N -> NormalMode.D [order 2] : [(VTQD_GearShiftPosn_enum == ENUM_GEARSHIFTPOSN_D && VFUN_EVDriveReady_flg ...
        |   && !VSCP_GearFlashInd_flg && !VTQD_DMSLossLimitGear_flg && !VDMM_DTCDMSRCIncorrect_flg...
        |   && ((VINP_BrkSwOn_flg && VINP_VehSpd_kph<=KTQD_GearShiftDAllowSpd_kph &&...
        |  abs(VINP_TMSpd_rpm) <= KTQD_GearShiftDAllowTMSpd_rpm)||...
        |   (VINP_VehSpd_kph > KTQD_GearShiftDAllowSpd_kph && ...
        |    VSCP_EVCU1VehActDrvDir_enum ~= ENUM_VEHACTDRVDIR_BACKWARD)))]
    (junction 380) -> (junction 382) : [(VTQD_ParkingPawlUnlockTimeOut_flg || VTQD_GearShiftPosn_enum == ENUM_GEARSHIFTPOSN_P)]
    AutoP -> (junction 380) [order 1]
    NormalMode.D -> AutoP [order 4] : [(VTQD_AutoPark_flg)]
    NormalMode.D -> (junction 88) [order 3] : [((VTQD_GearShiftPosn_enum == ENUM_GEARSHIFTPOSN_P)&&...
        | (VINP_VehSpd_kph<=KTQD_GearShiftPSpd_kph))]
    (junction 93) -> NormalMode.D : [(VTQD_GearShiftPosn_enum == ENUM_GEARSHIFTPOSN_D &&...
        |   VTQD_PTUnlock_flg && VPSA_IGNActive_flg)]
    AutoP -> NormalMode.D [order 2] : [(VTQD_PTUnlock_flg)]
    NormalMode.D -> NormalMode.R [order 1] : [(KTQD_GearShiftDRAllowSW_flg && ...
        |   VTQD_GearShiftPosn_enum == ENUM_GEARSHIFTPOSN_R &&...
        |   VINP_VehSpd_kph<=KTQD_GearShiftRAllowSpd_kph)]
    NormalMode.R -> NormalMode.D [order 1] : [(KTQD_GearShiftDRAllowSW_flg && ...
        |   VTQD_GearShiftPosn_enum == ENUM_GEARSHIFTPOSN_D &&...
        |   VINP_VehSpd_kph<=KTQD_GearShiftDAllowSpd_kph)]
    (junction 90) -> NormalMode.R
    NormalMode.R -> (junction 78) [order 3] : [ VTQD_GearShiftPosn_enum == ENUM_GEARSHIFTPOSN_N ...
        |   || (!VFUN_EVDriveReady_flg) || (VTQD_GearShiftPosn_enum == ENUM_GEARSHIFTPOSN_INVALID || ...
        |   VSCP_GearFlashInd_flg) || VDMM_DTCDMSRCIncorrect_flg || ...
        | (VTQD_DMSLossLimitGear_flg && VINP_VehSpd_kph<=KTQD_DMSLostTorqLimit_kph)]
    NormalMode.R -> (junction 89) [order 2] : [(VTQD_GearShiftPosn_enum == ENUM_GEARSHIFTPOSN_P)&&...
        | (VINP_VehSpd_kph<=KTQD_GearShiftPSpd_kph)]
    (junction 94) -> NormalMode.R : [(VTQD_GearShiftPosn_enum == ENUM_GEARSHIFTPOSN_R &&...
        |   VTQD_PTUnlock_flg && VPSA_IGNActive_flg)]
  (default) -> NormalMode
  NormalMode -> ADASMode : [VTQD_ExtShiftAvail_flg && VINP_ADASShftPosnReqA_flg]
  ADASMode -> NormalMode : [!VTQD_ExtShiftAvail_flg]
  data: VTQD_GearShiftPosn_enum input; VINP_VehSpd_kph input; VINP_ParkingPawlLock_flg input; VINP_BrkSwOn_flg input; task_time_s input; VTQD_GearActualPosn_enum output uint8; ENUM_GEARACTUALPOSN_N parameter; ENUM_GEARSHIFTPOSN_R parameter; ENUM_GEARSHIFTPOSN_D parameter; ENUM_GEARSHIFTPOSN_N parameter; ENUM_GEARACTUALPOSN_D parameter; ENUM_GEARACTUALPOSN_R parameter; TRUE parameter; FALSE parameter; ENUM_GEARACTUALPOSN_P parameter; ENUM_GEARSHIFTPOSN_P parameter; VTQD_ParkingPawlLockTime_s local single; VTQD_ParkingPawlPwrOn_flg output boolean; VTQD_ParkingPawlEnable_flg output boolean; VTQD_PTLock_flg local boolean; VTQD_ParkingPawlLockTimeOut_flg local boolean; VFUN_EVDriveReady_flg input; VTQD_PTUnlock_flg local boolean; VTQD_ParkingPawLockTime_s local single; VPSA_IGNActive_flg input; VTQD_InitializeTime_s local single; VTQD_RNDTrig_flg input; VTQD_AutoPark_flg input; VTQD_ADASModeDisact_flg input; VTQD_ParkingPawUnlockTime_s local single; VTQD_ParkingPawlUnlockTimeOut_flg local boolean; VTQD_ParkingPawlUnlockTime_s local single; VTQD_ExtShiftAvail_flg input; VINP_ADASShftPosnReqA_flg input; ENUM_GEARSHIFTPOSN_INVALID parameter; VSCP_EVCU1VehActDrvDir_enum input; VSCP_GearFlashInd_flg input; ENUM_VEHACTDRVDIR_BACKWARD parameter; ENUM_VEHACTDRVDIR_FORWARD parameter; VTQD_DMSLossLimitGear_flg input; VINP_TMSpd_rpm input; VDMM_DTCDMSRCIncorrect_flg input; VINP_ParkBrakeSW_flg input; KTQD_DMSLostTorqLimit_kph parameter; KTQD_GearShiftDAllowSpd_kph parameter; KTQD_GearShiftDAllowTMSpd_rpm parameter; KTQD_GearShiftDRAllowSW_flg parameter; KTQD_GearShiftPSpd_kph parameter; KTQD_GearShiftRAllowSpd_kph parameter; KTQD_GearShiftRAllowTMSpd_rpm parameter; KTQD_InitializeWaitTime_s parameter; KTQD_InitializeWaitTime4ADAS_s parameter; KTQD_RotateShiftMaxTime_s parameter

== stateflow chart tqd/TQD/Input_Convert/Input Signal Convert/Engineering Mode Enable Flasher/Chart ==
  state init
    en:
    time_cnt = ZERO_INT;
    ON_flg = TRUE;
    OFF_flg = FALSE;
    out = FALSE;
    CycleCnt_cnt = FALSE;
  state OFF
    en:
    out = FALSE;
    time_cnt = ZERO_INT;
    OFF -> (junction 38) [order 1]
    (junction 38) -> OFF : {time_cnt = time_cnt + ZERO_INT;}
  state ON
    en:
    out = TRUE;
    time_cnt = ZERO_INT;
    du:
    time_cnt = time_cnt + ONE_INT;
  state WAIT
    en:
    out = FALSE;
    time_cnt = ZERO_INT;
    du:
    time_cnt = time_cnt + ONE_INT;
  (default) -> init
  init -> (junction 57)
  (junction 57) -> ON : [ON_flg && VSCP_FlasherEn_flg]
  OFF -> (junction 46) [order 2] : [time_cnt > OFF_cnt]
  (junction 46) -> (junction 47) : {time_cnt = ZERO_INT;
      |  ON_flg = TRUE;
      |  OFF_flg = FALSE;
      |  CycleCnt_cnt = CycleCnt_cnt +ONE_INT;}
  (junction 47) -> ON : [ON_flg]
  ON -> (junction 44) : [time_cnt > ON_cnt]
  (junction 44) -> (junction 42) : {time_cnt = ZERO_INT;
      |  ON_flg = FALSE;
      |  OFF_flg = TRUE;}
  (junction 42) -> OFF : [OFF_flg]
  OFF -> (junction 66) [order 1] : [time_cnt > OFF_cnt && CycleCnt_cnt >= Cycle_cnt]
  (junction 66) -> WAIT : {time_cnt = ZERO_INT;}
  (junction 62) -> ON : {time_cnt = ZERO_INT;
      |  ON_flg = TRUE;
      |  OFF_flg = FALSE;
      |  CycleCnt_cnt = ZERO_INT;}
  WAIT -> (junction 62) : [time_cnt >= WAIT_cnt && VSCP_FlasherEn_flg]
  data: ON_cnt input; OFF_cnt input; WAIT_cnt input; Cycle_cnt input; out output boolean; time_cnt local uint8; OFF_flg local boolean; ON_flg local boolean; CycleCnt_cnt local uint8; VSCP_FlasherEn_flg input; FALSE parameter; TRUE parameter; ONE_INT parameter; ZERO_INT parameter
